simulink model "Model_FC_v12_Edit_for_Full_Scale_Fuel_Cell_GAS - Copy"  (R2017a)
settings: Solver=VariableStepAuto  StartTime=0  StopTime=20  FixedStep=0.01  MaxStep=1e-4  RelTol=1e-3  EnableMultiTasking=on
undefined symbols (not defined in the file or in its folder): sigbuilder_block
libraries: powerlib x9, simulink x6, fl_lib x5, nesl_utility x3, powerlib_meascontrol x1
(part 3 of 3)

== system Model_FC_v12_Edit_for_Full_Scale_Fuel_Cell_GAS - Copy/Integral Controller1 ==
  Output Voltage : Inport
  Add : Sum  Inputs=-+
  Add1 : Sum  Inputs=+-
  Amplifier : Gain  Gain=100
  Constant2 : Constant  Value=220
  Integrator : simulink/Continuous/PID Controller  Controller=I  TimeDomain=Continuous-time  SampleTime=-1  IntegratorMethod=Forward Euler  FilterMethod=Forward Euler  Form=Parallel  UseFilter=on  ControllerParametersSource=internal  P=1  I=40000  D=0  N=100  InitialConditionSource=internal  InitialConditionForIntegrator=0  InitialConditionForFilter=0  ExternalReset=falling  LimitOutput=off  UpperSaturationLimit=inf  LowerSaturationLimit=-inf  LinearizeAsGain=on  AntiWindupMode=none  Kb=1  TrackingMode=off  Kt=1  PParamMin=[]  PParamMax=[]  IParamMin=[]  IParamMax=[]  DParamMin=[]  DParamMax=[]  NParamMin=[]  NParamMax=[]  KbParamMin=[]  KbParamMax=[]  KtParamMin=[]  KtParamMax=[]  POutMin=[]  POutMax=[]  IOutMin=[]  IOutMax=[]  DOutMin=[]  DOutMax=[]  NOutMin=[]  NOutMax=[]  KbOutMin=[]  KbOutMax=[]  KtOutMin=[]  KtOutMax=[]  IntegratorOutMin=[]  IntegratorOutMax=[]  FilterOutMin=[]  FilterOutMax=[]  SumOutMin=[]  SumOutMax=[]  SumI1OutMin=[]  SumI1OutMax=[]  SumI2OutMin=[]  SumI2OutMax=[]  SumI3OutMin=[]  SumI3OutMax=[]  SumDOutMin=[]  SumDOutMax=[]  SaturationOutMin=[]  SaturationOutMax=[]  IntegratorContinuousStateAttributes=''  IntegratorStateMustResolveToSignalObject=off  IntegratorRTWStateStorageClass=Auto  FilterContinuousStateAttributes=''  FilterStateMustResolveToSignalObject=off  FilterRTWStateStorageClass=Auto  DifferentiatorICPrevScaledInput=0  DifferentiatorOutMin=[]  DifferentiatorOutMax=[]  InitialConditionSetting=State (most efficient)
  Pulse Generator2 : DiscretePulseGenerator  PulseType=Time based  Period=1/5e3  PulseWidth=73.23
  Relay : Relay
  Feedback Line : Outport
  wires:
  Output Voltage/1 -> Add/1
  Relay/1 -> Feedback Line/1
  Integrator/1 -> Add1/1
  Constant2/1 -> Add/2, Add1/2
  Add/1 -> Amplifier/1
  Amplifier/1 -> Integrator/1
  Add1/1 -> Relay/1
  Pulse Generator2/1 -> Integrator/2

== system Model_FC_v12_Edit_for_Full_Scale_Fuel_Cell_GAS - Copy/Load ==
  note: This Block models the Load Profile as dictated by the ship Resistance in the Nile River
  Signal : Inport
  Bus Selector : BusSelector  OutputSignals=Cell Output Voltage (V),Number Of Cells
  Current from Load profile of one day : Subsystem  Tag=STV Subsys  LoadFcn=sigbuilder_block('load');  StartFcn=sigbuilder_block('start');  StopFcn=sigbuilder_block('stop');  ClipboardFcn=sigbuilder_block('clipboard');  mask(Sigbuilder block){tuvar=[0:10]}
      mask help: Simulink:masks:SigbuilderBlock_MD
      mask init:
      | if ~strcmp(get_param(bdroot(gcbh),'SimulationStatus'),'stopped') tuvar = sigbuilder_block('maskInit'); end
      settings: CopyFcn=sigbuilder_block('copy');  DeleteFcn=sigbuilder_block('delete');  ModelCloseFcn=sigbuilder_block('modelClose');  PreSaveFcn=sigbuilder_block('preSave');  PauseFcn=sigbuilder_block('pause');  ContinueFcn=sigbuilder_block('continue');  NameChangeFcn=sigbuilder_block('namechange');  OpenFcn=sigbuilder_block('open',[403.5 117 550.5 359.25 ]);  CloseFcn=sigbuilder_block('close');
      mask Display: plot(0, 0, 100, 100,[2, 2, 32, 32, 2], [68, 8, 8, 68, 68],[32, 2], [38, 38], [32, 19, 2],[53, 60, 44], [32, 17, 17, 2],[16, 16, 31, 31]);txt = getActiveGroup(gcbh);text(2, 100, txt,'verticalAlignment', 'top');
  Product : Product
  Single day Variable Current : Subsystem  DialogController=hmiCreateDDGDialog  IsWebBlock=on  mask(MathWorksWebBlock){webBlockId=c4e3daab-8dab-4642-a272-c974aaedb1ac, webBlockType=sdiscope, ShowInitialText=on, HMISrcModelName=Model_FC_v12_Edit_for_Full_Scale_Fuel_Cell_GAS}
      mask prompts: webBlockId "WebBlock Id"; webBlockType "WebBlock Type"; HMISrcModelName "Source Model"
      mask Help: helpview([docroot '/mapfiles/simulink.map'], 'hmi_scope')
      mask Display:
      | if strcmp(get_param(bdroot(gcb),'BlockDiagramType'), 'library')
      |     image([(matlabroot) '/toolbox/simulink/hmi/icons/DashboardScope.png']);
      | end
  Total Output Voltage : Subsystem  DialogController=hmiCreateDDGDialog  IsWebBlock=on  mask(MathWorksWebBlock){webBlockId=81580c46-4ac5-4980-a5b4-9a4d2062d879, webBlockType=sdiscope, ShowInitialText=on, HMISrcModelName=Model_FC_v12_Edit_for_Full_Scale_Fuel_Cell_GAS}
      mask prompts: webBlockId "WebBlock Id"; webBlockType "WebBlock Type"; HMISrcModelName "Source Model"
      mask Help: helpview([docroot '/mapfiles/simulink.map'], 'hmi_scope')
      mask Display:
      | if strcmp(get_param(bdroot(gcb),'BlockDiagramType'), 'library')
      |     image([(matlabroot) '/toolbox/simulink/hmi/icons/DashboardScope.png']);
      | end
  Load Profile Current : Outport
  Total Output Voltage (V) : Outport  Port=2
  wires:
  Signal/1 -> Bus Selector/1
  Bus Selector/1 -> Product/1  "<Cell Output Voltage (V)>"
  Product/1 -> Total Output Voltage (V)/1  "Total Output Voltage (V)"
  Current from Load profile of one day/2(Signal 2) -> Load Profile Current/1  "Current from Load profile (Alex to Aswan)"
  Bus Selector/2 -> Product/2  "<Number Of Cells>"

== system Model_FC_v12_Edit_for_Full_Scale_Fuel_Cell_GAS - Copy/Signal Builder ==
  Demux : Demux  Tag=STV Demux  Outputs=1
  FromWs : FromWorkspace  Tag=STV FromWs  VariableName=tuvar  SampleTime=0
      SigBuilderData=|
      | common.afterFinalStr = 'Extrapolate'
      | common.sampleTime = 0
      | dataSet.timeRange = [0 10]
      | dataSet.name = 'Group 1'
      | sbobj.Groups.Name = 'Group 1'
      | sbobj.Groups.Signals.Name = 'Signal 1'
      | sbobj.Groups.Signals.XData = [0 0.09 10]
      | sbobj.Groups.Signals.YData = [1e-07 2.8e-05 2.8e-05]
  Signal 1 : Outport  Tag=STV Outport
  wires:
  Demux/1 -> Signal 1/1
  FromWs/1 -> Demux/1

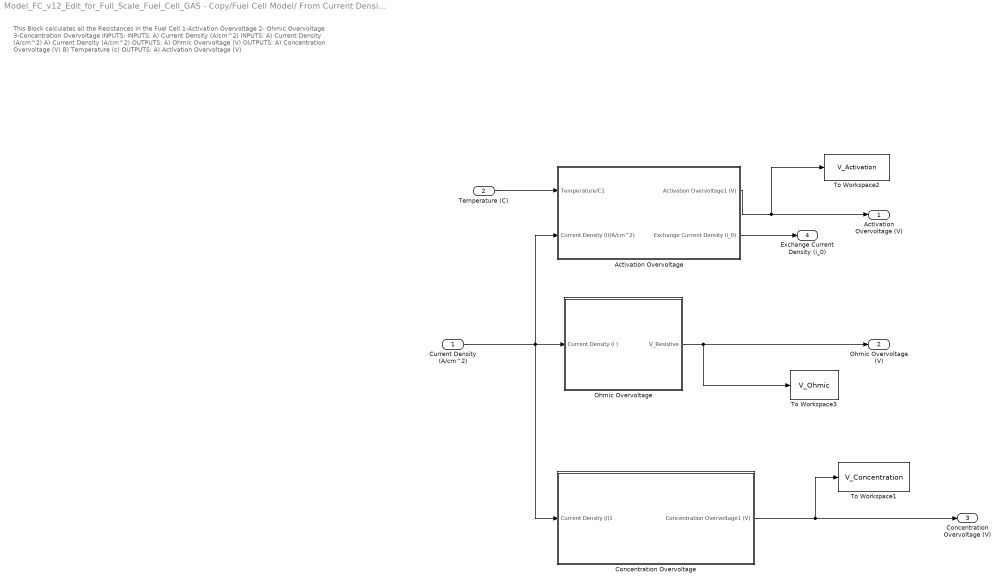
== system Model_FC_v12_Edit_for_Full_Scale_Fuel_Cell_GAS - Copy/Fuel Cell Model/ From Current Density (A//cm^2) To Overvoltages (V) ==
  note: This Block calculates all the Resistances in the Fuel Cell
      | 1-Activation Overvoltage 2- Ohmic Overvoltage 3-Concentration Overvoltage
      | INPUTS: INPUTS: A) Current Density (A/cm^2) INPUTS: A) Current Density (A/cm^2)
      | A) Current Density (A/cm^2) OUTPUTS: A) Ohmic Overvoltage (V) OUTPUTS: A) Concentration Overvoltage (V)
      | B) Temperature (c)
      |
      | OUTPUTS:
      | A) Activation Overvoltage (V)
  Current Density (A/cm^2) : Inport
  Temperature (C) : Inport  Port=2
  Activation Overvoltage : Subsystem
  Concentration Overvoltage : Subsystem
  Ohmic Overvoltage : Subsystem
  To Workspace1 : ToWorkspace  VariableName=V_Concentration  SampleTime=-1
      settings: Save2DSignal=2-D array (concatenate along first dimension)
  To Workspace2 : ToWorkspace  VariableName=V_Activation  SampleTime=-1
      settings: Save2DSignal=2-D array (concatenate along first dimension)
  To Workspace3 : ToWorkspace  VariableName=V_Ohmic  SampleTime=-1
      settings: Save2DSignal=2-D array (concatenate along first dimension)
  Activation Overvoltage (V) : Outport
  Ohmic Overvoltage (V) : Outport  Port=2
  Concentration Overvoltage (V) : Outport  Port=3
  Exchange Current Density (i_0) : Outport  Port=4
  wires:
  Temperature (C)/1 -> Activation Overvoltage/1(Temperature/C1)
  Current Density (A/cm^2)/1 -> Activation Overvoltage/2(Current Density (i)(A/cm^2)), Concentration Overvoltage/1(Current Density (i)1), Ohmic Overvoltage/1(Current Density (i ))
  Ohmic Overvoltage/1(V_Resistive) -> Ohmic Overvoltage (V)/1, To Workspace3/1
  Activation Overvoltage/1(Activation Overvoltage1 (V)) -> To Workspace2/1, Activation Overvoltage (V)/1
  Concentration Overvoltage/1("Concentration Overvoltage1 (V) ") -> To Workspace1/1, Concentration Overvoltage (V)/1
  Activation Overvoltage/2(Exchange Current Density (i_0)) -> Exchange Current Density (i_0)/1

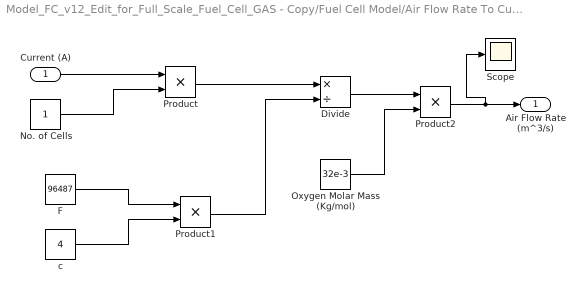
== system Model_FC_v12_Edit_for_Full_Scale_Fuel_Cell_GAS - Copy/Fuel Cell Model/Air Flow Rate To Current (A)1 ==
  Current (A) : Inport
  Divide : Product  Inputs=*/
  F : Constant  Value=96487
  No. of Cells : Constant
  Oxygen Molar Mass (Kg/mol) : Constant  Value=32e-3
  Product : Product
  Product1 : Product
  Product2 : Product
  Scope : Scope
  c : Constant  Value=4
  Air Flow Rate (m^3/s) : Outport
  wires:
  Current (A)/1 -> Product/1
  No. of Cells/1 -> Product/2
  Product/1 -> Divide/1
  F/1 -> Product1/1
  c/1 -> Product1/2
  Product1/1 -> Divide/2
  Divide/1 -> Product2/1
  Oxygen Molar Mass (Kg/mol)/1 -> Product2/2
  Product2/1 -> Scope/1, Air Flow Rate (m^3/s)/1

== system Model_FC_v12_Edit_for_Full_Scale_Fuel_Cell_GAS - Copy/Fuel Cell Model/Current Density A//cm^2 (Polarization Curve) ==
  Demux : Demux  Tag=STV Demux  Outputs=1
  FromWs : FromWorkspace  Tag=STV FromWs  VariableName=tuvar  SampleTime=0
      SigBuilderData=|
      | common.afterFinalStr = 'Extrapolate'
      | common.sampleTime = 0
      | dataSet.timeRange = [0 10]
      | dataSet.name = 'Group 1'
      | sbobj.Groups.Name = 'Group 1'
      | sbobj.Groups.Signals.Name = 'Signal 1'
      | sbobj.Groups.Signals.XData = [0 5 10]
      | sbobj.Groups.Signals.YData = [0.01 1.5 3]
  Signal 1 : Outport  Tag=STV Outport
  wires:
  Demux/1 -> Signal 1/1
  FromWs/1 -> Demux/1

== system Model_FC_v12_Edit_for_Full_Scale_Fuel_Cell_GAS - Copy/Fuel Cell Model/From Mass Flow Rates (kg//s) To Current Density (A//cm^2) ==
  note: The function of this block is to convert the input Hydrogen Mass Flow rate (Kg/s) to Current (A) then divide it by the Cell Area (cm^2) to get (Current Density) (A/cm^2)
      | which will be the input of several other blocks.
      | Inputs: a)Hydrogen Mass Flow Rate (kg/s) Outputs: Current Density (A/cm^2)
      | b)Number of Cells
      | c) Cell Area (cm^2)
  Hydrogen Flow Rate (kg/s) : Inport
  Cell Area (cm^2) : Inport  Port=2
  Number Of Cells : Inport  Port=3
  From Current (A) To Current Density (A/cm^2) : Subsystem
  Fuel Mass Flow Rate (kg/s) To Current (A) : Subsystem
  Current Density (A/cm^2) : Outport
  wires:
  Cell Area (cm^2)/1 -> From Current (A) To Current Density (A/cm^2)/2(Cell Area (cm^2))
  Fuel Mass Flow Rate (kg/s) To Current (A)/1(Current (A)) -> From Current (A) To Current Density (A/cm^2)/1(Nominal Current (A))
  Hydrogen Flow Rate (kg/s)/1 -> Fuel Mass Flow Rate (kg/s) To Current (A)/1(Hydrogen Flow Rate (kg/s))
  From Current (A) To Current Density (A/cm^2)/1(Current Density (A/cm^2)) -> Current Density (A/cm^2)/1  "Current density (A/cm^2)"
  Number Of Cells/1 -> Fuel Mass Flow Rate (kg/s) To Current (A)/2(Number Of Cells)  "Number Of Cells"

== system Model_FC_v12_Edit_for_Full_Scale_Fuel_Cell_GAS - Copy/Fuel Cell Model/From Pressures (atm) To Nernest Voltage (V) ==
  note: This Block calculates the Partial Pressures of Hydrogen and Oxygen (atm) from their pressures (atm) then uses these values to calculate the Nernest Voltage (V)
      |
      | INPUTS: A) Current Density (i) (A/cm^2) OUTPUTS 1: A) Oxygen Partial Pressure (atm) OUTPUTS 2: A) Nernest Voltage (V)
      | B) Absolute Hydrogen Pressure (atm) B) Water Saturation Pressure (atm)
      | C) Absolute Air Pressure (atm) C) Hydrogen Partial Pressure(atm)
      | D) Temperature (c)
  Current Density (i) : Inport
  Hydrogen Pressure (atm) : Inport  Port=2
  Air Pressure (atm) : Inport  Port=3
  Temperature (C) : Inport  Port=4
  From Absolute Pressure (atm) To Partial Pressures (atm) : Subsystem
  From Partial Pressures (atm) To Nernest Voltage (V) : Subsystem
  Oxygen Partial Pressure : Outport
  Nernest Voltage (V) : Outport  Port=2
  Water Pressure : Outport  Port=3
  wires:
  Temperature (C)/1 -> From Partial Pressures (atm) To Nernest Voltage (V)/4(Temperature/C), From Absolute Pressure (atm) To Partial Pressures (atm)/4(Temperature/C)
  From Absolute Pressure (atm) To Partial Pressures (atm)/1(Hydrogen Partial Pressure (pp_H2)) -> From Partial Pressures (atm) To Nernest Voltage (V)/1(Hydrogen Partial Pressure)
  Hydrogen Pressure (atm)/1 -> From Absolute Pressure (atm) To Partial Pressures (atm)/2(Hydrogen Pressure (P_H2))
  From Partial Pressures (atm) To Nernest Voltage (V)/1(Nernest Voltage1) -> Nernest Voltage (V)/1
  From Absolute Pressure (atm) To Partial Pressures (atm)/2(Oxygen Partial Pressure pp_O2) -> Oxygen Partial Pressure/1, From Partial Pressures (atm) To Nernest Voltage (V)/2(Oxygen Partial Pressure)
  From Absolute Pressure (atm) To Partial Pressures (atm)/3(Water Pressure) -> Water Pressure/1, From Partial Pressures (atm) To Nernest Voltage (V)/3(Water Pressure (P_H2O))
  Current Density (i)/1 -> From Absolute Pressure (atm) To Partial Pressures (atm)/1(Current Density (i ))
  Air Pressure (atm)/1 -> From Absolute Pressure (atm) To Partial Pressures (atm)/3(Air Pressure (P_air))

== system Model_FC_v12_Edit_for_Full_Scale_Fuel_Cell_GAS - Copy/Load/Current from Load profile of one day ==
  Demux : Demux  Tag=STV Demux  Outputs=2
  FromWs : FromWorkspace  Tag=STV FromWs  VariableName=tuvar  SampleTime=0
      SigBuilderData=|
      | common.afterFinalStr = 'Extrapolate'
      | common.sampleTime = 0
      | dataSet.timeRange = [0 300]
      | dataSet.name = 'Group 1'
      | sbobj.Groups.Name = 'Group 1'
      | sbobj.Groups.Signals(1).Name = 'Signal 1'
      | sbobj.Groups.Signals(1).XData = [0 2.75 2.75 5.75 5.75 10.98 10.98 24 24 24.6 24.6 27.61 27.61 30.61 30.61 33.73 33.73 36.73 48 48 52.19 52.19 55.19 55.19 59.38 59.38 62.38 72 72 84 84 96 96 108 108 120 120 132 132 144 144 146.76 146.76 147.76 147.76 156 156 168 168 175.76 175.76 176.76 176.76 180 180 192 192 204 204 216 216 216.76 216.76 217.76 217.76 228 228 240 240 244.83 244.83 300]
      | sbobj.Groups.Signals(1).YData = [145.4545455 145.4545455 0.01 0.01 145.4545455 145.4545455 0.01 0.01 195.4545455 195.4545455 486.3636364 486.3636364 0.01 0.01 404.5454545 404.5454545 0.01 0.01 0.01 486.3636364 486.3636364 0.01 0.01 486.3636364 486.3636364 0.01 0.01 0.01 463.6363636 463.6363636 0.01 0.01 463.6363636 463.6363636 0.01 0.01 463.6363636 463.6363636 0.01 0.01 463.6363636 463.6363636 0.01 0.01 463.6363636 463.6363636 0.01 0.01 463.6363636 463.6363636 0.01 0.01 463.6363636 463.6363636 0.01 0.01 463.6363636 463.6363636 0.01 0.01 463.6363636 463.6363636 0.01 0.01 463.6363636 463.6363636 0.01 0.01 463.6363636 463.6363636 0.01 0.01]
      | sbobj.Groups.Signals(2).Name = 'Signal 2'
      | sbobj.Groups.Signals(2).XData = [0 300]
      | sbobj.Groups.Signals(2).YData = [140 140]
      | sbobj.Groups.TimeRange = [0 300]
  Signal 1 : Outport  Tag=STV Outport
  Signal 2 : Outport  Tag=STV Outport  Port=2
  wires:
  Demux/1 -> Signal 1/1
  FromWs/1 -> Demux/1
  Demux/2 -> Signal 2/1

== system Model_FC_v12_Edit_for_Full_Scale_Fuel_Cell_GAS - Copy/Load/Single day Variable Current ==

== system Model_FC_v12_Edit_for_Full_Scale_Fuel_Cell_GAS - Copy/Load/Total Output Voltage ==

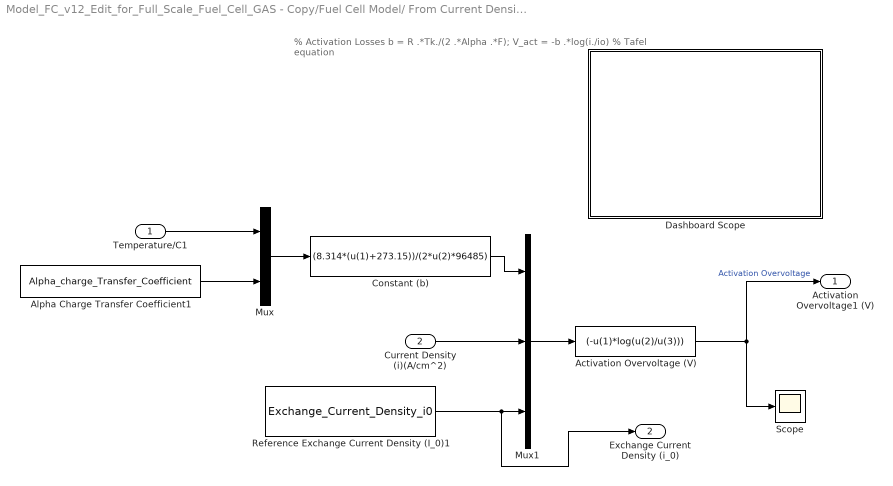
== system Model_FC_v12_Edit_for_Full_Scale_Fuel_Cell_GAS - Copy/Fuel Cell Model/ From Current Density (A//cm^2) To Overvoltages (V)/Activation Overvoltage ==
  note: % Activation Losses
      | b = R .*Tk./(2 .*Alpha .*F);
      | V_act = -b .*log(i./io) % Tafel equation
  Temperature/C1 : Inport
  Current Density (i)(A/cm^2) : Inport  Port=2
  Activation Overvoltage (V) : Fcn  Expr=(-u(1)*log(u(2)/u(3)))
  Alpha Charge Transfer Coefficient1 : Constant  Value=Alpha_charge_Transfer_Coefficient
  Constant (b) : Fcn  Expr=(8.314*(u(1)+273.15))/(2*u(2)*96485)
  Dashboard Scope : Subsystem  DialogController=hmiCreateDDGDialog  IsWebBlock=on  mask(MathWorksWebBlock){webBlockId=22b8d2ec-b744-4464-9b72-15b4b53948fb, webBlockType=sdiscope, ShowInitialText=on, HMISrcModelName=Model_FC_v12_Edit_for_Full_Scale_Fuel_Cell_GAS}
      mask prompts: webBlockId "WebBlock Id"; webBlockType "WebBlock Type"; HMISrcModelName "Source Model"
      mask Help: helpview([docroot '/mapfiles/simulink.map'], 'hmi_scope')
      mask Display:
      | if strcmp(get_param(bdroot(gcb),'BlockDiagramType'), 'library')
      |     image([(matlabroot) '/toolbox/simulink/hmi/icons/DashboardScope.png']);
      | end
  Mux : Mux  Inputs=2
  Mux1 : Mux  Inputs=3
  Reference Exchange Current Density (I_0)1 : Constant  Value=Exchange_Current_Density_i0
  Scope : Scope
  Activation Overvoltage1 (V) : Outport
  Exchange Current Density (i_0) : Outport  Port=2
  wires:
  Mux/1 -> Constant (b)/1
  Alpha Charge Transfer Coefficient1/1 -> Mux/2
  Temperature/C1/1 -> Mux/1
  Mux1/1 -> Activation Overvoltage (V)/1
  Constant (b)/1 -> Mux1/1
  Current Density (i)(A/cm^2)/1 -> Mux1/2
  Reference Exchange Current Density (I_0)1/1 -> Exchange Current Density (i_0)/1, Mux1/3
  Activation Overvoltage (V)/1 -> Activation Overvoltage1 (V)/1, Scope/1  "Activation Overvoltage"

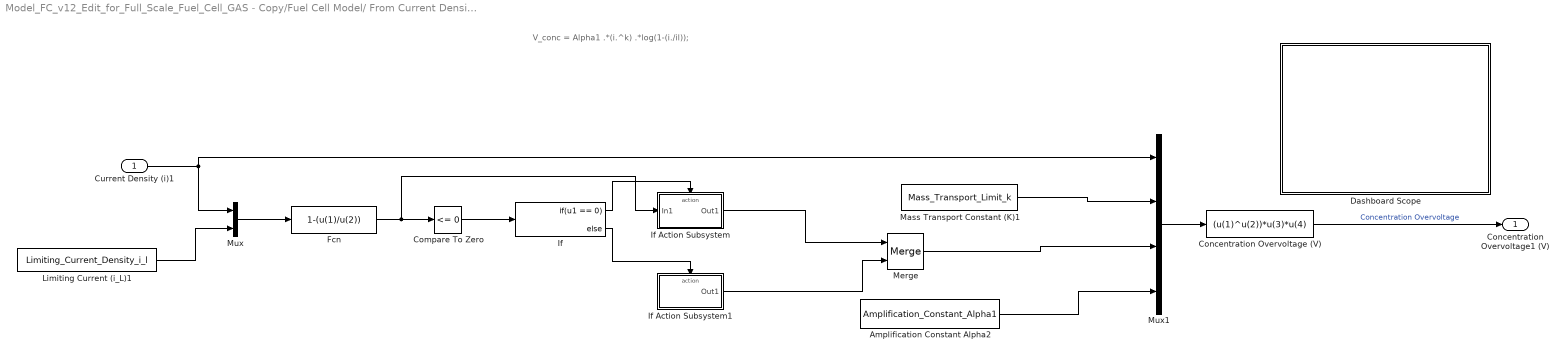
== system Model_FC_v12_Edit_for_Full_Scale_Fuel_Cell_GAS - Copy/Fuel Cell Model/ From Current Density (A//cm^2) To Overvoltages (V)/Concentration Overvoltage ==
  note: V_conc = Alpha1 .*(i.^k) .*log(1-(i./il));
  Current Density (i)1 : Inport
  Amplification Constant Alpha2 : Constant  Value=Amplification_Constant_Alpha1
  Compare To Zero : simulink/Logic and Bit Operations/Compare To Zero  relop=<=  OutDataTypeStr=boolean
  Concentration Overvoltage (V) : Fcn  Expr=(u(1)^u(2))*u(3)*u(4)
  Dashboard Scope : Subsystem  DialogController=hmiCreateDDGDialog  IsWebBlock=on  mask(MathWorksWebBlock){webBlockId=564ecfdb-cb30-4ab8-9f97-8672f30b7fa2, webBlockType=sdiscope, ShowInitialText=on, HMISrcModelName=Model_FC_v12_Edit_for_Full_Scale_Fuel_Cell_GAS}
      mask prompts: webBlockId "WebBlock Id"; webBlockType "WebBlock Type"; HMISrcModelName "Source Model"
      mask Help: helpview([docroot '/mapfiles/simulink.map'], 'hmi_scope')
      mask Display:
      | if strcmp(get_param(bdroot(gcb),'BlockDiagramType'), 'library')
      |     image([(matlabroot) '/toolbox/simulink/hmi/icons/DashboardScope.png']);
      | end
  Fcn : Fcn  Expr=1-(u(1)/u(2))
  If : If  IfExpression=u1 == 0
  If Action Subsystem : Subsystem  TreatAsAtomicUnit=on
  If Action Subsystem1 : Subsystem  TreatAsAtomicUnit=on
  Limiting Current (i_L)1 : Constant  Value=Limiting_Current_Density_i_l
  Mass Transport Constant (K)1 : Constant  Value=Mass_Transport_Limit_k
  Merge : Merge  InitialOutput=1
  Mux : Mux  Inputs=2
  Mux1 : Mux
  "Concentration Overvoltage1 (V) " : Outport
  wires:
  If/1 -> If Action Subsystem/Action
  If/2 -> If Action Subsystem1/Action
  If Action Subsystem/1(Out1) -> Merge/1
  If Action Subsystem1/1(Out1) -> Merge/2
  Compare To Zero/1 -> If/1
  Mux/1 -> Fcn/1
  Limiting Current (i_L)1/1 -> Mux/2
  Fcn/1 -> If Action Subsystem/1(In1), Compare To Zero/1
  Mux1/1 -> Concentration Overvoltage (V)/1
  Current Density (i)1/1 -> Mux1/1, Mux/1
  Mass Transport Constant (K)1/1 -> Mux1/2
  Merge/1 -> Mux1/3
  Amplification Constant Alpha2/1 -> Mux1/4
  Concentration Overvoltage (V)/1 -> "Concentration Overvoltage1 (V) "/1  "Concentration Overvoltage"

== system Model_FC_v12_Edit_for_Full_Scale_Fuel_Cell_GAS - Copy/Fuel Cell Model/ From Current Density (A//cm^2) To Overvoltages (V)/Ohmic Overvoltage ==
  Current Density (i ) : Inport
  Constant : Constant  Value=-1
  Dashboard Scope : Subsystem  DialogController=hmiCreateDDGDialog  IsWebBlock=on  mask(MathWorksWebBlock){webBlockId=c0b798d8-aea7-4029-a856-156eb00102c5, webBlockType=sdiscope, ShowInitialText=on, HMISrcModelName=Model_FC_v12_Edit_for_Full_Scale_Fuel_Cell_GAS}
      mask prompts: webBlockId "WebBlock Id"; webBlockType "WebBlock Type"; HMISrcModelName "Source Model"
      mask Help: helpview([docroot '/mapfiles/simulink.map'], 'hmi_scope')
      mask Display:
      | if strcmp(get_param(bdroot(gcb),'BlockDiagramType'), 'library')
      |     image([(matlabroot) '/toolbox/simulink/hmi/icons/DashboardScope.png']);
      | end
  Internal Resistance (r) : Constant  Value=Internal_Resistance_r
  V_Resistive1 : Product  Inputs=3
  V_Resistive : Outport
  wires:
  Constant/1 -> V_Resistive1/3
  Internal Resistance (r)/1 -> V_Resistive1/2
  Current Density (i )/1 -> V_Resistive1/1
  V_Resistive1/1 -> V_Resistive/1  "Ohmic Overvoltage (V)"

== system Model_FC_v12_Edit_for_Full_Scale_Fuel_Cell_GAS - Copy/Fuel Cell Model/From Mass Flow Rates (kg//s) To Current Density (A//cm^2)/From Current (A) To Current Density (A//cm^2) ==
  note: i=I/A
      | where i=Current Density (A/cm^2)
      | I= Current (A)
      | A=Cell Area (cm^2)
  Nominal Current (A) : Inport
  Cell Area (cm^2) : Inport  Port=2
  Divide : Product  Inputs=*/
  Current Density (A/cm^2) : Outport
  wires:
  Nominal Current (A)/1 -> Divide/1
  Cell Area (cm^2)/1 -> Divide/2
  Divide/1 -> Current Density (A/cm^2)/1

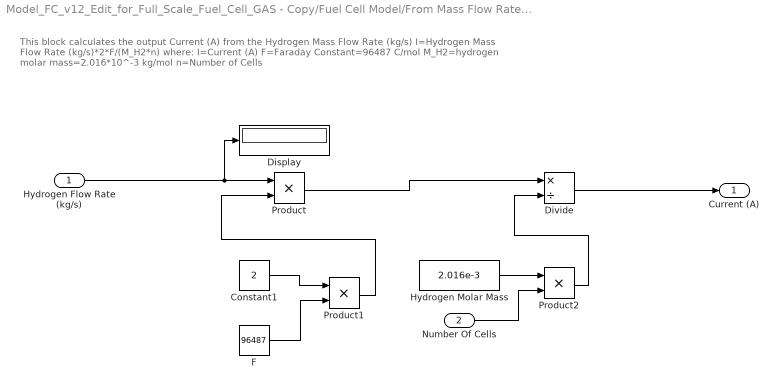
== system Model_FC_v12_Edit_for_Full_Scale_Fuel_Cell_GAS - Copy/Fuel Cell Model/From Mass Flow Rates (kg//s) To Current Density (A//cm^2)/Fuel Mass Flow Rate (kg//s) To Current (A) ==
  note: This block calculates the output Current (A) from the Hydrogen Mass Flow Rate (kg/s)
      | I=Hydrogen Mass Flow Rate (kg/s)*2*F/(M_H2*n)
      | where: I=Current (A)
      | F=Faraday Constant=96487 C/mol
      | M_H2=hydrogen molar mass=2.016*10^-3 kg/mol
      | n=Number of Cells
  Hydrogen Flow Rate (kg/s) : Inport
  Number Of Cells : Inport  Port=2
  Constant1 : Constant  Value=2
  Display : Display
  Divide : Product  Inputs=*/
  F : Constant  Value=96487
  Hydrogen Molar Mass : Constant  Value=2.016e-3
  Product : Product
  Product1 : Product
  Product2 : Product
  Current (A) : Outport
  wires:
  F/1 -> Product1/2
  Constant1/1 -> Product1/1
  Product1/1 -> Product/2
  Product/1 -> Divide/1
  Hydrogen Molar Mass/1 -> Product2/1
  Number Of Cells/1 -> Product2/2
  Product2/1 -> Divide/2
  Divide/1 -> Current (A)/1
  Hydrogen Flow Rate (kg/s)/1 -> Display/1, Product/1

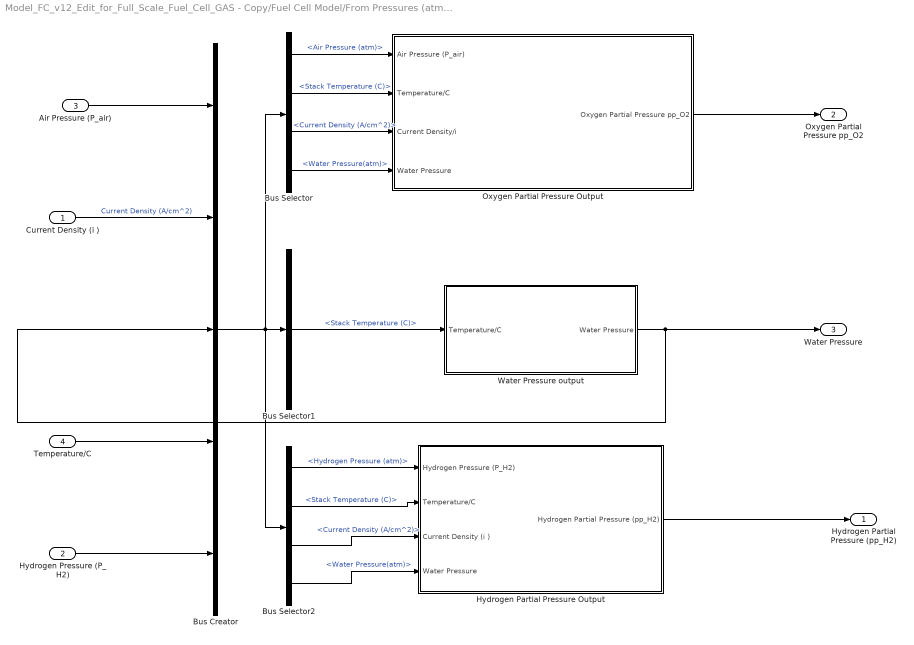
== system Model_FC_v12_Edit_for_Full_Scale_Fuel_Cell_GAS - Copy/Fuel Cell Model/From Pressures (atm) To Nernest Voltage (V)/From Absolute Pressure (atm) To Partial Pressures (atm) ==
  Current Density (i ) : Inport
  Hydrogen Pressure (P_H2) : Inport  Port=2
  Air Pressure (P_air) : Inport  Port=3
  Temperature/C : Inport  Port=4
  Bus Creator : BusCreator  Inputs=5
  Bus Selector : BusSelector  OutputSignals=Air Pressure (atm),Stack Temperature (C),Current Density (A/cm^2),Water Pressure(atm)
  Bus Selector1 : BusSelector  OutputSignals=Stack Temperature (C)
  Bus Selector2 : BusSelector  OutputSignals=Hydrogen Pressure (atm),Stack Temperature (C),Current Density (A/cm^2),Water Pressure(atm)
  Hydrogen Partial Pressure Output : Subsystem
  Oxygen Partial Pressure Output : Subsystem
  Water Pressure output : Subsystem
  Hydrogen Partial Pressure (pp_H2) : Outport
  Oxygen Partial Pressure pp_O2 : Outport  Port=2
  Water Pressure : Outport  Port=3
  wires:
  Water Pressure output/1(Water Pressure) -> Water Pressure/1, Bus Creator/3
  Air Pressure (P_air)/1 -> Bus Creator/1
  Oxygen Partial Pressure Output/1(Oxygen Partial Pressure pp_O2) -> Oxygen Partial Pressure pp_O2/1
  Hydrogen Partial Pressure Output/1(Hydrogen Partial Pressure (pp_H2)) -> Hydrogen Partial Pressure (pp_H2)/1
  Current Density (i )/1 -> Bus Creator/2  "Current Density (A/cm^2)"
  Temperature/C/1 -> Bus Creator/4
  Hydrogen Pressure (P_H2)/1 -> Bus Creator/5
  Bus Creator/1 -> Bus Selector2/1, Bus Selector/1, Bus Selector1/1
  Bus Selector/1 -> Oxygen Partial Pressure Output/1(Air Pressure (P_air))  "<Air Pressure (atm)>"
  Bus Selector/2 -> Oxygen Partial Pressure Output/2(Temperature/C)  "<Stack Temperature (C)>"
  Bus Selector/3 -> Oxygen Partial Pressure Output/3(Current Density/i)  "<Current Density (A/cm^2)>"
  Bus Selector/4 -> Oxygen Partial Pressure Output/4(Water Pressure)  "<Water Pressure(atm)>"
  Bus Selector1/1 -> Water Pressure output/1(Temperature/C)  "<Stack Temperature (C)>"
  Bus Selector2/1 -> Hydrogen Partial Pressure Output/1(Hydrogen Pressure (P_H2))  "<Hydrogen Pressure (atm)>"
  Bus Selector2/2 -> Hydrogen Partial Pressure Output/2(Temperature/C)  "<Stack Temperature (C)>"
  Bus Selector2/3 -> Hydrogen Partial Pressure Output/3(Current Density (i ))  "<Current Density (A/cm^2)>"
  Bus Selector2/4 -> Hydrogen Partial Pressure Output/4(Water Pressure)  "<Water Pressure(atm)>"

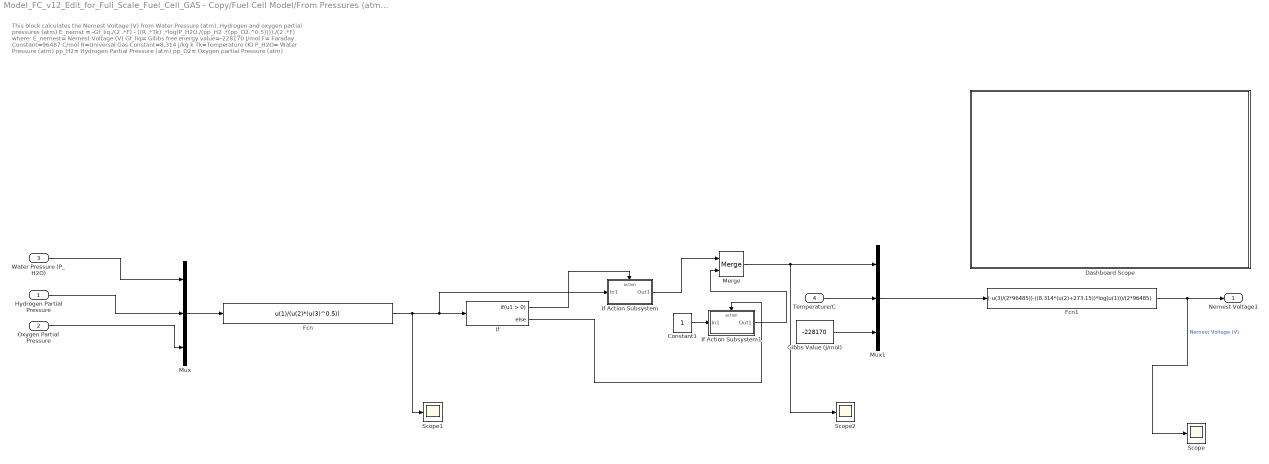
== system Model_FC_v12_Edit_for_Full_Scale_Fuel_Cell_GAS - Copy/Fuel Cell Model/From Pressures (atm) To Nernest Voltage (V)/From Partial Pressures (atm) To Nernest Voltage (V) ==
  note: This block calculates the Nernest Voltage (V) from Water Pressure (atm), Hydrogen and oxygen partial pressures (atm)
      | E_nernst = -Gf_liq./(2 .*F) - ((R .*Tk) .*log(P_H2O./(pp_H2 .*(pp_O2.^0.5))))./(2 .*F)
      | where: E_nernest= Nernest Voltage (V)
      | Gf_liq= Gibbs free energy value=-228170 J/mol
      | F= Faraday Constant=96487 C/mol
      | R=Universal Gas Constant=8.314 j/kg k
      | Tk=Temperature (K)
      | P_H2O= Water Pressure (atm)
      | pp_H2= Hydrogen Partial Pressure (atm)
      | pp_O2= Oxygen partial Pressure (atm)
  Hydrogen Partial Pressure : Inport
  Oxygen Partial Pressure : Inport  Port=2
  Water Pressure (P_H2O) : Inport  Port=3
  Temperature/C : Inport  Port=4
  Constant1 : Constant
  Dashboard Scope : Subsystem  DialogController=hmiCreateDDGDialog  IsWebBlock=on  mask(MathWorksWebBlock){webBlockId=5bd8e11a-4211-42d2-b432-bf660f2594da, webBlockType=sdiscope, ShowInitialText=on, HMISrcModelName=Model_FC_v12_Edit_for_Full_Scale_Fuel_Cell_GAS}
      mask prompts: webBlockId "WebBlock Id"; webBlockType "WebBlock Type"; HMISrcModelName "Source Model"
      mask Help: helpview([docroot '/mapfiles/simulink.map'], 'hmi_scope')
      mask Display:
      | if strcmp(get_param(bdroot(gcb),'BlockDiagramType'), 'library')
      |     image([(matlabroot) '/toolbox/simulink/hmi/icons/DashboardScope.png']);
      | end
  Fcn : Fcn  Expr=u(1)/(u(2)*(u(3)^0.5))
  Fcn1 : Fcn  Expr=(-u(3)/(2*96485))-((8.314*(u(2)+273.15))*log(u(1)))/(2*96485)
  Gibbs Value (J/mol) : Constant  Value=-228170
  If : If
  If Action Subsystem : Subsystem  TreatAsAtomicUnit=on
  If Action Subsystem1 : Subsystem  TreatAsAtomicUnit=on
  Merge : Merge
  Mux : Mux  Inputs=3
  Mux1 : Mux  Inputs=3
  Scope : Scope
  Scope1 : Scope
  Scope2 : Scope
  Nernest Voltage1 : Outport
  wires:
  Gibbs Value (J/mol)/1 -> Mux1/3
  Oxygen Partial Pressure/1 -> Mux/3
  If/1 -> If Action Subsystem/Action
  If Action Subsystem/1(Out1) -> Merge/1
  If/2 -> If Action Subsystem1/Action
  Constant1/1 -> If Action Subsystem1/1(In1)
  If Action Subsystem1/1(Out1) -> Merge/2
  Water Pressure (P_H2O)/1 -> Mux/1
  Hydrogen Partial Pressure/1 -> Mux/2
  Mux/1 -> Fcn/1
  Fcn/1 -> Scope1/1, If Action Subsystem/1(In1), If/1
  Merge/1 -> Scope2/1, Mux1/1
  Temperature/C/1 -> Mux1/2
  Mux1/1 -> Fcn1/1
  Fcn1/1 -> Scope/1, Nernest Voltage1/1  "Nernest Voltage (V)"

== system Model_FC_v12_Edit_for_Full_Scale_Fuel_Cell_GAS - Copy/Fuel Cell Model/ From Current Density (A//cm^2) To Overvoltages (V)/Activation Overvoltage/Dashboard Scope ==

== system Model_FC_v12_Edit_for_Full_Scale_Fuel_Cell_GAS - Copy/Fuel Cell Model/ From Current Density (A//cm^2) To Overvoltages (V)/Concentration Overvoltage/Dashboard Scope ==

== system Model_FC_v12_Edit_for_Full_Scale_Fuel_Cell_GAS - Copy/Fuel Cell Model/ From Current Density (A//cm^2) To Overvoltages (V)/Concentration Overvoltage/If Action Subsystem ==
  In1 : Inport
  Action Port : ActionPort  ActionType=then
  Math Function1 : Math  Operator=log  OutputSignalType=real  SaturateOnIntegerOverflow=on
  Out1 : Outport
  wires:
  In1/1 -> Math Function1/1
  Math Function1/1 -> Out1/1

== system Model_FC_v12_Edit_for_Full_Scale_Fuel_Cell_GAS - Copy/Fuel Cell Model/ From Current Density (A//cm^2) To Overvoltages (V)/Concentration Overvoltage/If Action Subsystem1 ==
  Action Port : ActionPort  ActionType=else
  Constant1 : Constant  Value=0
  Out1 : Outport
  wires:
  Constant1/1 -> Out1/1

== system Model_FC_v12_Edit_for_Full_Scale_Fuel_Cell_GAS - Copy/Fuel Cell Model/ From Current Density (A//cm^2) To Overvoltages (V)/Ohmic Overvoltage/Dashboard Scope ==

== system Model_FC_v12_Edit_for_Full_Scale_Fuel_Cell_GAS - Copy/Fuel Cell Model/From Pressures (atm) To Nernest Voltage (V)/From Absolute Pressure (atm) To Partial Pressures (atm)/Hydrogen Partial Pressure Output ==
  note: This block calculates the Hydrogen partial Pressure (pp_H2)(atm)
      | pp_H2 = 0.5 .*((P_H2)./(exp(1.653 .*i./(Tk.^1.334)))-P_H2O)
      | where: pp_H2= Hydrogen Partial Pressure (atm)
      | i=Current Density (A/cm^2)
      | Tk= Temperature in Kelvin
      | P_H2O= Water pressure (atm)
  Hydrogen Pressure (P_H2) : Inport
  Temperature/C : Inport  Port=2
  Current Density (i ) : Inport  Port=3
  Water Pressure : Inport  Port=4
  Dashboard Scope : Subsystem  DialogController=hmiCreateDDGDialog  IsWebBlock=on  mask(MathWorksWebBlock){webBlockId=ddeef619-4d6d-4ce8-b4bd-8db147ec0074, webBlockType=sdiscope, ShowInitialText=on, HMISrcModelName=Model_FC_v12_Edit_for_Full_Scale_Fuel_Cell_GAS}
      mask prompts: webBlockId "WebBlock Id"; webBlockType "WebBlock Type"; HMISrcModelName "Source Model"
      mask Help: helpview([docroot '/mapfiles/simulink.map'], 'hmi_scope')
      mask Display:
      | if strcmp(get_param(bdroot(gcb),'BlockDiagramType'), 'library')
      |     image([(matlabroot) '/toolbox/simulink/hmi/icons/DashboardScope.png']);
      | end
  Fcn : Fcn  Expr=0.5*((u(1))/(exp(1.653*u(2)/((u(3)+273.15)^1.334)))-u(4))
  Mux : Mux
  Scope : Scope
  Hydrogen Partial Pressure (pp_H2) : Outport
  wires:
  Water Pressure/1 -> Mux/4
  Temperature/C/1 -> Mux/3
  Current Density (i )/1 -> Scope/1, Mux/2
  Hydrogen Pressure (P_H2)/1 -> Mux/1
  Mux/1 -> Fcn/1
  Fcn/1 -> Hydrogen Partial Pressure (pp_H2)/1  "Hydrogen Partial Pressure (pp_H2)"

== system Model_FC_v12_Edit_for_Full_Scale_Fuel_Cell_GAS - Copy/Fuel Cell Model/From Pressures (atm) To Nernest Voltage (V)/From Absolute Pressure (atm) To Partial Pressures (atm)/Oxygen Partial Pressure Output ==
  note: This block calculates the Oxygen Partial Pressure (atm)
      | pp_O2 = (P_air./exp(4.192 .*i/(Tk.^1.334)))-P_H2O
      |
      | where: pp_O2= Oxygen Partial Pressure (atm)
      | P_air= Air Pressure (atm)
      | i= Current Density (A/cm^2)
      | Tk= Temperature (K)
      | P_H2O=Water Pressure (atm)
  Air Pressure (P_air) : Inport
  Temperature/C : Inport  Port=2
  Current Density/i : Inport  Port=3
  Water Pressure : Inport  Port=4
  Dashboard Scope : Subsystem  DialogController=hmiCreateDDGDialog  IsWebBlock=on  mask(MathWorksWebBlock){webBlockId=34d7efc1-0742-4b26-9118-642359a02322, webBlockType=sdiscope, ShowInitialText=on, HMISrcModelName=Model_FC_v12_Edit_for_Full_Scale_Fuel_Cell_GAS}
      mask prompts: webBlockId "WebBlock Id"; webBlockType "WebBlock Type"; HMISrcModelName "Source Model"
      mask Help: helpview([docroot '/mapfiles/simulink.map'], 'hmi_scope')
      mask Display:
      | if strcmp(get_param(bdroot(gcb),'BlockDiagramType'), 'library')
      |     image([(matlabroot) '/toolbox/simulink/hmi/icons/DashboardScope.png']);
      | end
  Fcn : Fcn  Expr=(u(1)/exp(4.192 *u(2)/((u(3)+273.15)^1.334)))-u(4)
  Mux : Mux
  Oxygen Partial Pressure pp_O2 : Outport
  wires:
  Current Density/i/1 -> Mux/2
  Water Pressure/1 -> Mux/4
  Temperature/C/1 -> Mux/3
  Air Pressure (P_air)/1 -> Mux/1
  Mux/1 -> Fcn/1
  Fcn/1 -> Oxygen Partial Pressure pp_O2/1  "Oxygen Partial Pressure pp_O2 (atm)"

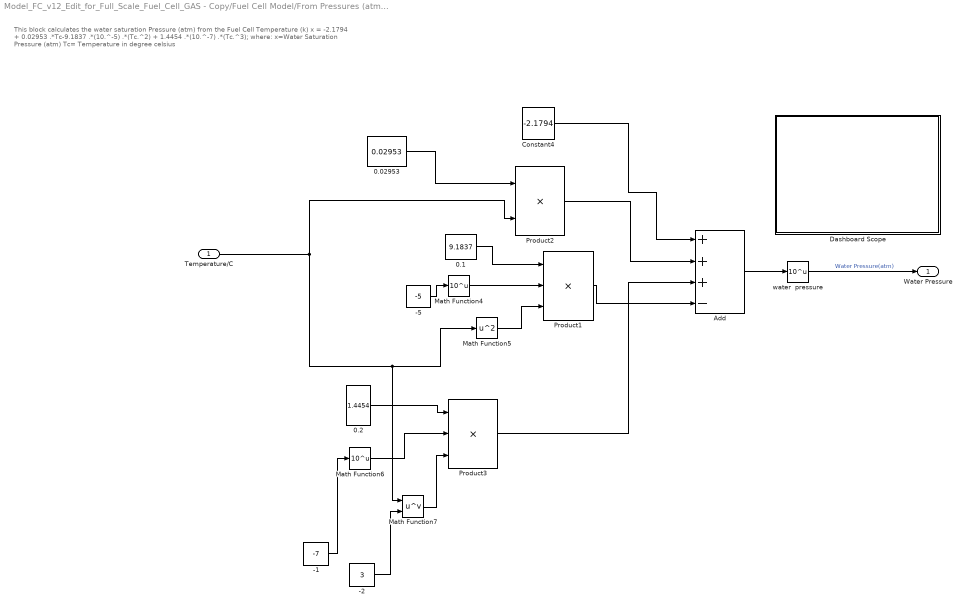
== system Model_FC_v12_Edit_for_Full_Scale_Fuel_Cell_GAS - Copy/Fuel Cell Model/From Pressures (atm) To Nernest Voltage (V)/From Absolute Pressure (atm) To Partial Pressures (atm)/Water Pressure output ==
  note: This block calculates the water saturation Pressure (atm) from the Fuel Cell Temperature (k)
      | x = -2.1794 + 0.02953 .*Tc-9.1837 .*(10.^-5) .*(Tc.^2) + 1.4454 .*(10.^-7) .*(Tc.^3);
      | where: x=Water Saturation Pressure (atm)
      | Tc= Temperature in degree celsius
  Temperature/C : Inport
  -1 : Constant  Value=-7
  -2 : Constant  Value=3
  -5 : Constant  Value=-5
  0.02953 : Constant  Value=0.02953
  0.1 : Constant  Value=9.1837
  0.2 : Constant  Value=1.4454
  Add : Sum  Inputs=+++-
  Constant4 : Constant  Value=-2.1794
  Dashboard Scope : Subsystem  DialogController=hmiCreateDDGDialog  IsWebBlock=on  mask(MathWorksWebBlock){webBlockId=75a5c32c-eec0-415c-91e1-99486c1b84a0, webBlockType=sdiscope, ShowInitialText=on, HMISrcModelName=Model_FC_v12_Edit_for_Full_Scale_Fuel_Cell_GAS}
      mask prompts: webBlockId "WebBlock Id"; webBlockType "WebBlock Type"; HMISrcModelName "Source Model"
      mask Help: helpview([docroot '/mapfiles/simulink.map'], 'hmi_scope')
      mask Display:
      | if strcmp(get_param(bdroot(gcb),'BlockDiagramType'), 'library')
      |     image([(matlabroot) '/toolbox/simulink/hmi/icons/DashboardScope.png']);
      | end
  Math Function4 : Math  Operator=10^u  SaturateOnIntegerOverflow=on
  Math Function5 : Math  Operator=square  SaturateOnIntegerOverflow=on
  Math Function6 : Math  Operator=10^u  SaturateOnIntegerOverflow=on
  Math Function7 : Math  Operator=pow  SaturateOnIntegerOverflow=on
  Product1 : Product  Inputs=3
  Product2 : Product
  Product3 : Product  Inputs=3
  "water  pressure " : Math  Operator=10^u  SaturateOnIntegerOverflow=on
  Water Pressure : Outport
  wires:
  Add/1 -> "water  pressure "/1
  0.2/1 -> Product3/1
  Math Function7/1 -> Product3/3
  "water  pressure "/1 -> Water Pressure/1  "Water Pressure(atm)"
  0.02953/1 -> Product2/1
  0.1/1 -> Product1/1
  -5/1 -> Math Function4/1
  Math Function4/1 -> Product1/2
  -1/1 -> Math Function6/1
  Temperature/C/1 -> Product2/2, Math Function5/1, Math Function7/1
  Math Function5/1 -> Product1/3
  -2/1 -> Math Function7/2
  Product2/1 -> Add/2
  Product3/1 -> Add/3
  Math Function6/1 -> Product3/2
  Constant4/1 -> Add/1
  Product1/1 -> Add/4

== system Model_FC_v12_Edit_for_Full_Scale_Fuel_Cell_GAS - Copy/Fuel Cell Model/From Pressures (atm) To Nernest Voltage (V)/From Partial Pressures (atm) To Nernest Voltage (V)/Dashboard Scope ==

== system Model_FC_v12_Edit_for_Full_Scale_Fuel_Cell_GAS - Copy/Fuel Cell Model/From Pressures (atm) To Nernest Voltage (V)/From Partial Pressures (atm) To Nernest Voltage (V)/If Action Subsystem ==
  In1 : Inport
  Action Port : ActionPort  ActionType=then
  Out1 : Outport
  wires:
  In1/1 -> Out1/1

== system Model_FC_v12_Edit_for_Full_Scale_Fuel_Cell_GAS - Copy/Fuel Cell Model/From Pressures (atm) To Nernest Voltage (V)/From Partial Pressures (atm) To Nernest Voltage (V)/If Action Subsystem1 ==
  In1 : Inport
  Action Port : ActionPort  ActionType=else
  Out1 : Outport
  wires:
  In1/1 -> Out1/1

== system Model_FC_v12_Edit_for_Full_Scale_Fuel_Cell_GAS - Copy/Fuel Cell Model/From Pressures (atm) To Nernest Voltage (V)/From Absolute Pressure (atm) To Partial Pressures (atm)/Hydrogen Partial Pressure Output/Dashboard Scope ==

== system Model_FC_v12_Edit_for_Full_Scale_Fuel_Cell_GAS - Copy/Fuel Cell Model/From Pressures (atm) To Nernest Voltage (V)/From Absolute Pressure (atm) To Partial Pressures (atm)/Oxygen Partial Pressure Output/Dashboard Scope ==

== system Model_FC_v12_Edit_for_Full_Scale_Fuel_Cell_GAS - Copy/Fuel Cell Model/From Pressures (atm) To Nernest Voltage (V)/From Absolute Pressure (atm) To Partial Pressures (atm)/Water Pressure output/Dashboard Scope ==
